simulink model "motor_pid_model"  (R2017a)
settings: Solver=VariableStepAuto  StartTime=0.0  StopTime=1  FixedStep=1e-4  RelTol=1e-4
InitFcn:
  | Tw=0.01;     %Ancho de Ventana
  | ppv=20;      %Pulsos por vuelta
  | Ts=1e-4;     %Tiempo de muestreo
  | 
  | Kp=0.001;
  | Kd=0.02;
  | Ki=0.4;
  | h=Tw;
  | N=100;
  | 
  | % Los valores de num, den se obtienen de punto_2.m
  | % Fueron hardcodeados por comodidad.
  | 
  | num = [0 0.7770 0];
  | den = [1.0000 -0.9918 -0.0061];
settings Model: Creator=Martin  LastModifiedBy=Alan

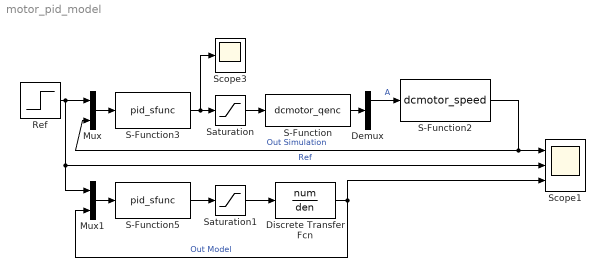
== system motor_pid_model ==
  Demux : Demux  Outputs=2
  Discrete Transfer Fcn : DiscreteTransferFcn  Numerator=num  Denominator=den
  Mux : Mux  Inputs=2
  Mux1 : Mux  Inputs=2
  Ref : Step  Time=0.2  After=4200  SampleTime=Ts
  S-Function : S-Function  FunctionName=dcmotor_qenc  Parameters=ppv  SFunctionDeploymentMode=off  EnableBusSupport=off
  S-Function2 : S-Function  FunctionName=dcmotor_speed  Parameters=Ts,ppv,Tw  SFunctionDeploymentMode=off  EnableBusSupport=off
  S-Function3 : S-Function  FunctionName=pid_sfunc  Parameters=Kp,Kd,Ki,h,N  SFunctionDeploymentMode=off  EnableBusSupport=off
  S-Function5 : S-Function  FunctionName=pid_sfunc  Parameters=Kp,Kd,Ki,h,N  SFunctionDeploymentMode=off  EnableBusSupport=off
  Saturation : Saturate  UpperLimit=30  LowerLimit=-30
  Saturation1 : Saturate  UpperLimit=30  LowerLimit=-30
  Scope1 : Scope  NumInputPorts=3
  Scope3 : Scope
  wires:
  Ref/1 -> Mux1/1, Scope1/2, Mux/1  "Ref"
  S-Function/1 -> Demux/1
  Demux/1 -> S-Function2/1  "A"
  S-Function2/1 -> Scope1/1, Mux/2  "Out Simulation"
  Mux/1 -> S-Function3/1
  Saturation/1 -> S-Function/1
  S-Function3/1 -> Scope3/1, Saturation/1
  S-Function5/1 -> Saturation1/1
  Saturation1/1 -> Discrete Transfer Fcn/1
  Mux1/1 -> S-Function5/1
  Discrete Transfer Fcn/1 -> Scope1/3, Mux1/2  "Out Model"
